simulink model "sim_projectile"  (Simulink 8.1)
settings: Solver=ode45  StartTime=0.0  StopTime=50  MaxStep=0.01  RelTol=1e-3
undefined symbols (not defined in the file or in its folder): magnitude
libraries: simulink x2
settings Model: Creator=Rudi  LastModifiedBy=rudi
settings OptimizationCC: InitFltsAndDblsToZero=on
settings DebuggingCC: SaveWithParameterizedLinksMsg=none  StrictBusMsg=Warning
settings SFSimCC: SimParseCustomCode=off
settings GRTTargetCC: TargetFcnLib=ansi_tfl_tmw.mat

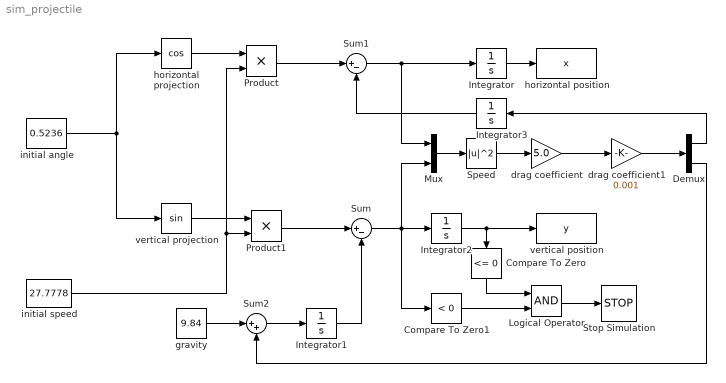
== system sim_projectile ==
  Compare To Zero : simulink/Logic and Bit Operations/Compare To Zero  relop=<=  OutDataTypeStr=boolean  ZeroCross=off
  Compare To Zero1 : simulink/Logic and Bit Operations/Compare To Zero  relop=<  OutDataTypeStr=boolean  ZeroCross=off
  Demux : Demux  Outputs=2
  Integrator{,1..3} (4 alike) : Integrator
  Logical Operator : Logic  AllPortsSameDT=off  OutDataTypeStr=boolean
  Mux : Mux  Inputs=2
  Product : Product  RndMeth=Zero
  Product1 : Product  RndMeth=Zero
  Speed : Math  Operator=magnitude^2  SaturateOnIntegerOverflow=on
  Stop Simulation : Stop
  Sum : Sum  Inputs=|+-
  Sum1 : Sum  Inputs=|+-
  Sum2 : Sum  Inputs=|++
  drag coefficient : Gain  Gain=5.0
  drag coefficient1 : Gain  Gain=0.001
  gravity : Constant  Value=9.84
  horizontal position : ToWorkspace  VariableName=x  SampleTime=-1
  horizontal projection : Trigonometry  Operator=cos
  initial angle : Constant  Value=0.5236
  initial speed : Constant  Value=27.7778
  vertical position : ToWorkspace  VariableName=y  SampleTime=-1
  vertical projection : Trigonometry
  wires:
  initial angle/1 -> horizontal projection/1, vertical projection/1
  horizontal projection/1 -> Product/1
  vertical projection/1 -> Product1/1
  initial speed/1 -> Product1/2, Product/2
  Integrator/1 -> horizontal position/1
  Sum/1 -> Integrator2/1, Mux/2, Compare To Zero1/1
  Integrator2/1 -> vertical position/1, Compare To Zero/1
  Compare To Zero/1 -> Logical Operator/1
  Logical Operator/1 -> Stop Simulation/1
  Compare To Zero1/1 -> Logical Operator/2
  Sum1/1 -> Integrator/1, Mux/1
  Product1/1 -> Sum/1
  Product/1 -> Sum1/1
  Integrator1/1 -> Sum/2
  Integrator3/1 -> Sum1/2
  gravity/1 -> Sum2/1
  Sum2/1 -> Integrator1/1
  Mux/1 -> Speed/1
  Speed/1 -> drag coefficient/1
  Demux/1 -> Integrator3/1
  Demux/2 -> Sum2/2
  drag coefficient/1 -> drag coefficient1/1
  drag coefficient1/1 -> Demux/1
